simulink model "quartercarmodelwithvaryingdamping"  (R2025a)
settings: Solver=VariableStepAuto  StartTime=0.0  StopTime=10.0  RelTol=1e-3
undefined symbols (not defined in the file): c_com, c_re, k1, k2, mc, ms, v
settings Model: Creator=krishDragneel  LastModifiedBy=krishDragneel

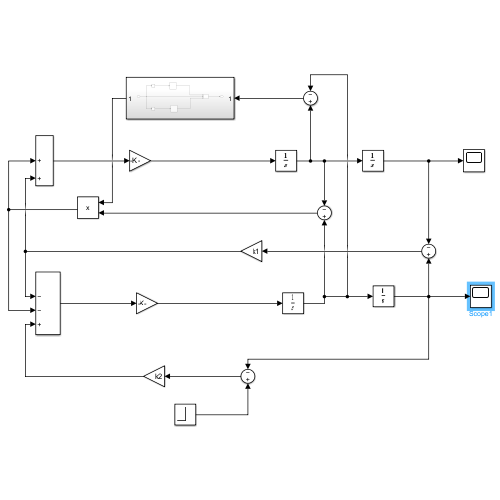
[thumbnail: Simulink's stored preview of the top-level diagram]
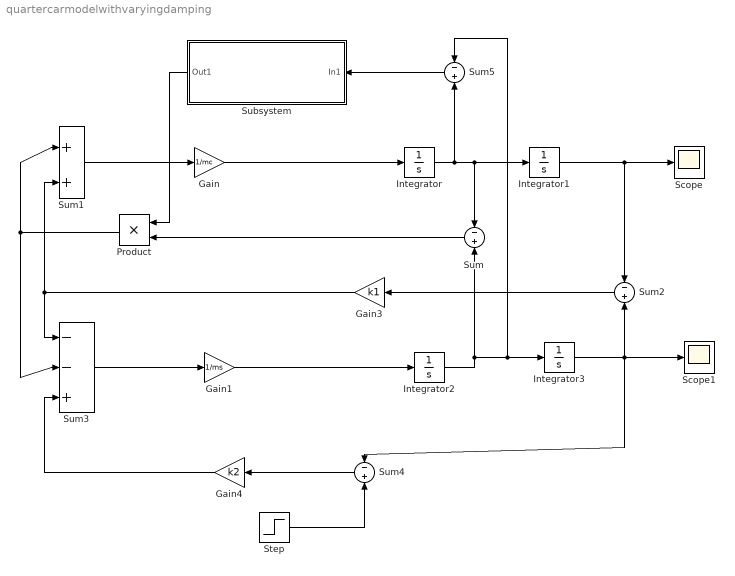
== system quartercarmodelwithvaryingdamping ==
  Gain : Gain  Gain=1/mc
  Gain1 : Gain  Gain=1/ms
  Gain3 : Gain  Gain=k1
  Gain4 : Gain  Gain=k2
  Integrator{,1..3} (4 alike) : Integrator
  Product : Product
  Scope : Scope
      settings: ActiveDisplayYMinimum=-5.1852029753195223  ActiveDisplayYMaximum=46.666826777875713
  Scope1 : Scope
      settings: ActiveDisplayYMinimum=-6.9981075547345641  ActiveDisplayYMaximum=62.982967992611094
  Step : Step  After=30  SampleTime=0
  Subsystem : Subsystem
  Sum{,2,4..5} (4 alike) : Sum  Inputs=-+
  Sum1 : Sum  Inputs=|++
  Sum3 : Sum  Inputs=|--+
  wires:
  Integrator/1 -> Integrator1/1, Sum/1, Sum5/2
  Sum2/1 -> Gain3/1
  Integrator2/1 -> Sum5/1, Integrator3/1, Sum/2
  Integrator3/1 -> Sum4/1, Scope1/1, Sum2/2
  Sum4/1 -> Gain4/1
  Gain4/1 -> Sum3/3
  Integrator1/1 -> Sum2/1, Scope/1
  Sum3/1 -> Gain1/1
  Sum/1 -> Product/2
  Gain1/1 -> Integrator2/1
  Sum1/1 -> Gain/1
  Gain3/1 -> Sum1/2, Sum3/1
  Gain/1 -> Integrator/1
  Step/1 -> Sum4/2
  Sum5/1 -> Subsystem/1(In1)
  Subsystem/1(Out1) -> Product/1
  Product/1 -> Sum3/2, Sum1/1

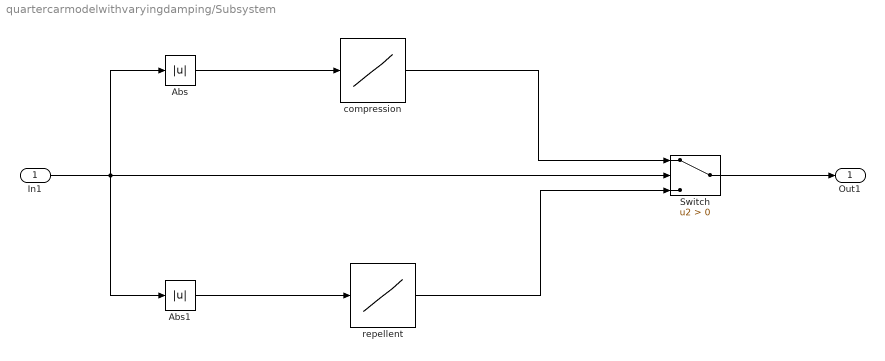
== system quartercarmodelwithvaryingdamping/Subsystem ==
  In1 : Inport
  Abs : Abs  SaturateOnIntegerOverflow=off
  Abs1 : Abs  SaturateOnIntegerOverflow=off
  Switch : Switch  Criteria=u2 > Threshold  SaturateOnIntegerOverflow=off  InputSameDT=off
  compression : Lookup_n-D  NumberOfTableDimensions=1  BreakpointsForDimension1=v  Table=c_com  InternalRulePriority=Speed  RndMeth=Simplest
  repellent : Lookup_n-D  NumberOfTableDimensions=1  BreakpointsForDimension1=v  Table=c_re  InternalRulePriority=Speed  RndMeth=Simplest
  Out1 : Outport
  wires:
  In1/1 -> Switch/2, Abs1/1, Abs/1
  Abs/1 -> compression/1
  Abs1/1 -> repellent/1
  compression/1 -> Switch/1
  repellent/1 -> Switch/3
  Switch/1 -> Out1/1
